simulink model "SEPotencia_ControlTiempoReal_PBL"  (R2021a)
settings: Solver=ode3  StartTime=0.0  StopTime=SimulationTime  FixedStep=StepTime  RelTol=1e-4
PreLoadFcn:
  | clear all;
  | clc;
  | mex Moduladora.c;
  | 
  | %% Parametros Simulacion
  | StepTime = 1.6e-6;
  | SimulationTime = 2;
  | ConstanteTiempo = 159e-6;
  | 
  | %% Motor
  | P = 186.5;
  | Vff = 220;
  | FrecFundamental =  60;
  | VelocidadMotor = 1800;
  | ParPolos = 2;
  | Rs = 11.05;
  | Ls = 3.164e-3;
  | Rr = 6.11;
  | Lr = Ls;
  | Lm = 293.94e-3;
  | Inercia = 0.0005;
  | Tm = 0.05;
  | 
  | %% Consigna Velocidad
  | velocidadInicial=1725/VelocidadMotor;
  | velocidadStepTime = 1;
  | velocidadFinal = 1725/VelocidadMotor;
  | 
  | %% Inversor
  | Vdc = 311;
  | Tconmut = 200e-6;
  | FrecConmut=1/Tconmut;
  | RampaAceleracion = 500/0.2/VelocidadMotor;
  | TiempoMuerto = 4e-6;
  | Kc=1/6;
  | 
  | %% DSP
  | NBits = 12;
  | OffSet = 0.1;
  | PWMSelect = 1; % Pot <= 0, DSP > 0
  | 
  | %Control
  | Kp = 200;
  | Ki = 0;
  | Kd = 0;
  | Control = 1; % Control PI <= 0, Control Step > 0
  | Activar3Armonico = 1; % 3Armonico Activo > 0, 3Armonico Desativado <= 0
  | OverCurrentLimit = 10;
  | VffPU = Vff/Vdc/0.6124;
  | if (Activar3Armonico > 0)
  |     limiteSuperior = 1.154;
  |     if (VffPU > limiteSuperior)
  |         VffPU = limiteSuperior;
  |     end
  | else
  |     limiteSuperior = 1;
  |     if (VffPU > limiteSuperior)
  |         VffPU = limiteSuperior;
  |     end
  | end
  | RelacionVF = (VffPU-0)/(1-0);
  | PI_Num = 3.14159265359;
InitFcn:
  | clear all;
  | clc;
  | mex Moduladora.c;
  | 
  | %% Parametros Simulacion
  | StepTime = 1.6e-6;
  | SimulationTime = 2;
  | ConstanteTiempo = 159e-6;
  | 
  | %% Motor
  | P = 186.5;
  | Vff = 220;
  | FrecFundamental =  60;
  | VelocidadMotor = 1800;
  | ParPolos = 2;
  | Rs = 11.05;
  | Ls = 3.164e-3;
  | Rr = 6.11;
  | Lr = Ls;
  | Lm = 293.94e-3;
  | Inercia = 0.0005;
  | Tm = 0.05;
  | 
  | %% Consigna Velocidad
  | velocidadInicial=600/VelocidadMotor;
  | velocidadStepTime = 1;
  | velocidadFinal = 850/VelocidadMotor;
  | 
  | %% Inversor
  | Vdc = 311;
  | Tconmut = 200e-6;
  | FrecConmut=1/Tconmut;
  | RampaAceleracion = 500/0.2/VelocidadMotor;
  | TiempoMuerto = 4e-6;
  | Kc=1/6;
  | 
  | %% DSP
  | NBits = 12;
  | OffSet = 0.1;
  | PWMSelect = 1; % Pot <= 0, DSP > 0
  | 
  | %Control
  | Kp = 5;
  | Ki = 150;
  | Kd = 0;
  | Control = 1; % Control PI <= 0, Control Step > 0
  | Activar3Armonico = 1; % 3Armonico Activo > 0, 3Armonico Desativado <= 0
  | OverCurrentLimit = 10;
  | VffPU = Vff/Vdc/0.6124;
  | if (Activar3Armonico > 0)
  |     limiteSuperior = 1.154;
  |     if (VffPU > limiteSuperior)
  |         VffPU = limiteSuperior;
  |     end
  | else
  |     limiteSuperior = 1;
  |     if (VffPU > limiteSuperior)
  |         VffPU = limiteSuperior;
  |     end
  | end
  | RelacionVF = (VffPU-0)/(1-0);
  | PI_Num = 3.14159265359;
undefined symbols (not defined in the file or in its folder): DiscIntNeverNeededParam
libraries: spsDCVoltageSourceLib x2, spsFirstOrderFilterLib x2, spsRMSLib x2, spsAsynchronousMachineSIUnitsLib x1, pid_lib x1, spsOnDelayLib x1, spsTriangleGeneratorLib x1, spsGroundLib x1, eeGeneralControl x1, spsTwoLevelConverterLib x1, spsThreePhaseVIMeasurementLib x1, spspowerguiLib x1
settings Model: Creator=The MathWorks, Inc.  LastModifiedBy=Yago
settings SolverCC: AlgebraicLoopSolver=TrustRegion  SolverResetMethod=Robust
settings DataIOCC: ReturnWorkspaceOutputs=off
settings OptimizationCC: LifeSpan=inf
settings DebuggingCC: ReadBeforeWriteMsg=DisableAll  WriteAfterWriteMsg=DisableAll  WriteAfterReadMsg=DisableAll  MultiTaskDSMMsg=none  UnconnectedInputMsg=none  UnconnectedOutputMsg=none  UnconnectedLineMsg=none  SFUnexpectedBacktrackingDiag=warning  SFNoUnconditionalDefaultTransitionDiag=warning  SFExecutionAtInitializationDiag=none  SFMachineParentedDataDiag=warning  ArithmeticOperatorsInVariantConditions=warning
settings ModelReferenceCC: UpdateModelReferenceTargets=IfOutOfDate
settings SFSimCC: SFSimEcho=off  SimUseLocalCustomCode=off  CustomCodeUndefinedFunction=UseInterfaceOnly
settings RTWCC: RTWUseLocalCustomCode=off
settings CodeAppCC: StateflowObjectComments=on
settings GRTTargetCC: TargetLangStandard=C89/C90 (ANSI)
settings ConfigComp: CovMetricSettings=dw  CovSaveCumulativeToWorkspaceVar=on  CovSaveSingleToWorkspaceVar=on  CovExternalEMLEnable=off
settings SimscapeCC: SimscapeNormalizeSystem=off  SimscapeNominalValues={1, 'bar'; 1, 'cm^3/s'; 1, 'bar*kg/s'; 1, 'kJ/kg'; 1, 'kW'; }

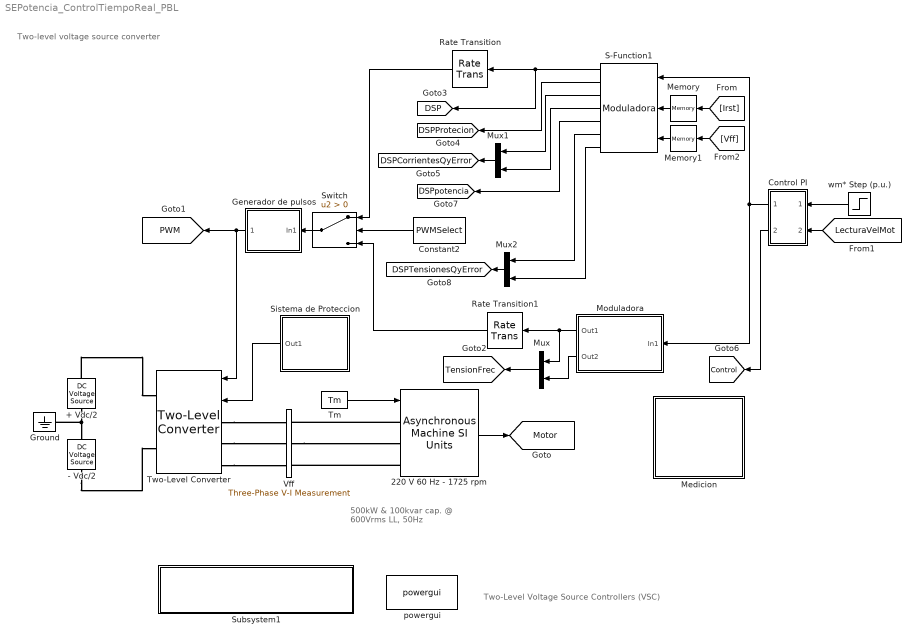
== system SEPotencia_ControlTiempoReal_PBL ==
  note: Two-level voltage source converter
  note: 500kW & 100kvar cap.
      | @ 600Vrms LL, 50Hz
  note: Two-Level Voltage Source Controllers (VSC)
  + Vdc/2 : spsDCVoltageSourceLib/DC Voltage Source  Amplitude=Vdc/2  Measurements=None
  - Vdc/2 : spsDCVoltageSourceLib/DC Voltage Source  Amplitude=Vdc/2  Measurements=None
  220 V 60 Hz - 1725 rpm : spsAsynchronousMachineSIUnitsLib/Asynchronous Machine SI Units  RotorType=Squirrel-cage  PresetModel=No  MechanicalLoad=Torque Tm  ShowDetailedParameters=on  ReferenceFrame=Stationary  Units=SI  MeasurementBus=on  NominalParameters=[ P, Vff, FrecFundamental ]  VoltageRatio=1  Stator="[ Rs  Ls ]"  Rotor="[ Rr  Lr ]"  Cage1=[ 0.022 0.226/377]  Cage2=[ 0.022 0.226/377]  Lm=Lm  Mechanical="[ Inercia  0 ParPolos]"  PolePairs=2  InitialConditions="[ 1,0   0,0,0   0,0,0 ]"  SimulateSaturation=off  Saturation=[14.03593122, 27.81365428, 53.79336849, 72.68890987, 97.98006896, 148.6815601, 215.7428561, 302.9841135, 428.7778367 ; 230, 322, 414, 460, 506, 552, 598, 644, 690]  LoadFlowParameters=0  TsPowergui=0  TsBlock=-1  IterativeModel=Trapezoidal non iterative  IterativeDiscreteModel=Trapezoidal non iterative  Pmec=0
      settings: AttributesFormatString=\n
  Constant2 : Constant  Value=PWMSelect
  Control PI : Subsystem  TreatAsAtomicUnit=on  SystemSampleTime=Tconmut
  Generador de pulsos : Subsystem  SystemSampleTime=Tconmut
  Ground : spsGroundLib/Ground  LConnTagsString=a
  Medicion : Subsystem
  Memory : Memory  LinearizeAsDelay=on
  Memory1 : Memory  LinearizeAsDelay=on
  Moduladora : Subsystem  TreatAsAtomicUnit=on  SystemSampleTime=Tconmut
  Mux : Mux  Inputs=2
  Mux1 : Mux  Inputs=2
  Mux2 : Mux  Inputs=2
  Rate Transition : RateTransition
  Rate Transition1 : RateTransition
  S-Function1 : S-Function  FunctionName=Moduladora  Parameters=Tconmut NBits OffSet RampaAceleracion FrecFundamental FrecConmut Kc limiteSuperior Activar3Armonico OverCurrentLimit Vdc Vff  SFunctionDeploymentMode=off  EnableBusSupport=off
  Sistema de Proteccion : Subsystem
  Subsystem1 : Subsystem  ClipboardFcn=""
      settings: OpenFcn=|
      | t=ScopeData1.time;
      | FundFreq=50;
      | MaxFreq=5000;
      | FFTDATA = power_fftscope(ScopeData1);
      | FFTDATA.input=1;
      | FFTDATA.signal=1;
      | FFTDATA.startTime='last';
      | FFTDATA.cycles=1;
      | FFTDATA.fundamental=FundFreq;
      | FFTDATA.maxFrequency=MaxFreq;
      | FFTDATA.THDmaxFrequency=MaxFreq;
      | FFTDATA.THDbase='fund';
      | power_fftscope(FFTDATA);
      | xlabel('Ia prim 6-pulse');
      | ScreenS=get(0,'Screensize');
      | x0=ScreenS(3); y0=ScreenS(4);
      | PositionParam=[x0/26 y0/3.1 x0/3.8 y0/2.5];
      | set(gcf,'Position',PositionParam);
      | axis([0 5000 0 35])
      | grid
      | FFTDATA = power_fftscope(ScopeData1);
      | FFTDATA.input=3;
      | FFTDATA.signal=1;
      | FFTDATA.startTime='last';
      | FFTDATA.cycles=1;
      | FFTDATA.fundamental=FundFreq;
      | FFTDATA.maxFrequency=MaxFreq;
      | FFTDATA.THDmaxFrequency=MaxFreq;
      | FFTDATA.THDbase='fund';
      | power_fftscope(FFTDATA);
      | xlabel('Ia prim 12-pulse');
      | ScreenS=get(0,'Screensize');
      | x0=ScreenS(3); y0=ScreenS(4);
      | PositionParam=[x0/3.2 y0/3.1 x0/3.8 y0/2.5];
      | set(gcf,'Position',PositionParam);
      | axis([0 5000 0 35])
      | grid
      mask Display: disp('Compare VSC''s\nLine-Line Voltage')
  Switch : Switch  Criteria=u2 > Threshold
  Tm : Constant  Value=Tm
  Two-Level Converter : spsTwoLevelConverterLib/Two-Level Converter  ModelType=Switching devices  Ron=1e-3  Rs=1e6  Cs=inf  Vforward=[0,0]  Ron_Diode=1e-3  Rs_Diode=1e6  Cs_Diode=inf  Vf_Diode=1e-3  Rs_CurrentSource=inf
      settings: SourceProductBaseCode=PS
  Vff : spsThreePhaseVIMeasurementLib/Three-Phase V-I Measurement  VoltageMeasurement=phase-to-phase  SetLabelV=on  LabelV=Vff  Vpu=off  VpuLL=off  CurrentMeasurement=yes  SetLabelI=on  LabelI=Irst  Ipu=off  Pbase=1e3  Vbase=380  OutputType=Magnitude  PhasorSimulation=off  PSBequivalent=0
  powergui : spspowerguiLib/powergui  Priority=1  SimulationMode=Discrete  SampleTime=StepTime  frequency=60  Iterations=50  frequencyindice=0  Pbase=100e6  ErrMax=1e-4  UnitsV=kV  UnitsW=MW  buscounter=0  FunctionMessages=off  echomessages=off  EnableUseOfTLC=off  CurrentSourceSwitches=off  DisableSnubberDevices=off  DisableRonSwitches=off  DisableVfSwitches=off  DisplayEquations=off  AutomaticDiscreteSolvers=off  SolverType=Tustin/Backward Euler (TBE)  Interpol=off  ExternalGateDelay=off  methode=off  Ts=100  x0status=blocks  SPID=off  SwTol=0  HookPort=off  NonlinearTolerance=1e-4  nMaxIteration=100  ContinueOnMaxIteration=off  RestoreLinks=warning  ResistiveCurrentMeasurement=off  Frange=[0:2:500]  Ylog=off  Xlog=on  ShowGrid=off  save=off  variable=ZData  structure=0  ZoomFFT=off  StartTime=0.0  cycles=1  DisplayStyle=1  fundamental=60  FreqAxis=off  MaxFrequency=1000  frequencyindicesteady=1  RmsSteady=1  display=off
  wm* Step (p.u.) : Step  Time=velocidadStepTime  Before=velocidadInicial  After=velocidadFinal  SampleTime=StepTime
  tag scope: Control=global, DSP=global, DSPCorrientesQyError=global, DSPProtecion=global, DSPTensionesQyError=global, DSPpotencia=global, Motor=global, PWM=global, TensionFrec=global
  wires:
  S-Function1/1 -> [DSP], Rate Transition/1
  Constant2/1 -> Switch/2
  Memory/1 -> S-Function1/2
  Tm/1 -> 220 V 60 Hz - 1725 rpm/1
  220 V 60 Hz - 1725 rpm/1 -> [Motor]
  Rate Transition/1 -> Switch/1
  Switch/1 -> Generador de pulsos/1(In1)
  Moduladora/1(Out1) -> Rate Transition1/1, Mux/1
  Generador de pulsos/1("  ") -> [PWM], Two-Level Converter/1
  Mux/1 -> [TensionFrec]
  Moduladora/2(Out2) -> Mux/2
  Rate Transition1/1 -> Switch/3
  S-Function1/2 -> [DSPProtecion]
  Control PI/1(Out1) -> S-Function1/1, Moduladora/1(In1)
  wm* Step (p.u.)/1 -> Control PI/1(In1)
  Sistema de Proteccion/1(Out1) -> Two-Level Converter/2
  Mux1/1 -> [DSPCorrientesQyError]
  S-Function1/3 -> Mux1/1
  S-Function1/4 -> Mux1/2
  [Irst] -> Memory/1
  [LecturaVelMot] -> Control PI/2(In2)
  Control PI/2(Out2) -> [Control]
  [Vff] -> Memory1/1
  Memory1/1 -> S-Function1/3
  S-Function1/5 -> [DSPpotencia]
  S-Function1/6 -> Mux2/1
  S-Function1/7 -> Mux2/2
  Mux2/1 -> [DSPTensionesQyError]
  connections:
  Two-Level Converter/LConn2 -- Vff/LConn2
  220 V 60 Hz - 1725 rpm/LConn3 -- Vff/RConn3
  Two-Level Converter/LConn3 -- Vff/LConn3
  Two-Level Converter/LConn1 -- Vff/LConn1
  220 V 60 Hz - 1725 rpm/LConn1 -- Vff/RConn1
  + Vdc/2/RConn1 -- Two-Level Converter/RConn1
  - Vdc/2/LConn1 -- Two-Level Converter/RConn2
  + Vdc/2/LConn1 -- - Vdc/2/RConn1 -- Ground/LConn1
  Vff/RConn2 -- 220 V 60 Hz - 1725 rpm/LConn2

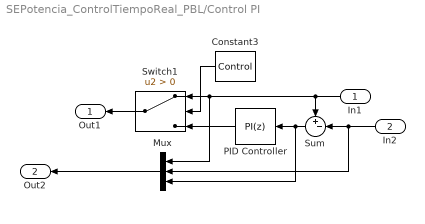
== system SEPotencia_ControlTiempoReal_PBL/Control PI ==
  In1 : Inport
  In2 : Inport  Port=2
  Constant3 : Constant  Value=Control
  Mux : Mux  Inputs=3
  PID Controller : pid_lib/PID Controller  Controller=PI  Form=Parallel  TimeDomain=Discrete-time  UseExternalTs=off  SampleTime=-1  IntegratorMethod=Trapezoidal  FilterMethod=Forward Euler  ControllerParametersSource=internal  P=Kp  I=1/Ki  D=Kd  UseFilter=on  N=100  TunerSelectOption=Transfer Function Based (PID Tuner App)  InitialConditionSource=internal  InitialConditionForIntegrator=0  InitialConditionForFilter=0  DifferentiatorICPrevScaledInput=0  ExternalReset=none  TrackingMode=off  Kt=1  LimitOutput=on  SatLimitsSource=internal  UpperSaturationLimit=1.5  LowerSaturationLimit=-1.5  LinearizeAsGain=on  AntiWindupMode=none  Kb=1  POutMin=[]  POutMax=[]  IOutMin=[]  IOutMax=[]  DOutMin=[]  DOutMax=[]  NOutMin=[]  NOutMax=[]  SumOutMin=[]  SumOutMax=[]  SaturationOutMin=[]  SaturationOutMax=[]  PParamMin=[]  PParamMax=[]  IParamMin=[]  IParamMax=[]  DParamMin=[]  DParamMax=[]  NParamMin=[]  NParamMax=[]  KbParamMin=[]  KbParamMax=[]  KtParamMin=[]  KtParamMax=[]  KbOutMin=[]  KbOutMax=[]  KtOutMin=[]  KtOutMax=[]  IntegratorOutMin=[]  IntegratorOutMax=[]  FilterOutMin=[]  FilterOutMax=[]  SumI1OutMin=[]  SumI1OutMax=[]  SumI2OutMin=[]  SumI2OutMax=[]  SumI3OutMin=[]  SumI3OutMax=[]  SumI4OutMin=[]  SumI4OutMax=[]  SumDOutMin=[]  SumDOutMax=[]  DifferentiatorOutMin=[]  DifferentiatorOutMax=[]  FilterDiffOutCoefMin=[]  FilterDiffOutCoefMax=[]  ReciprocalOutMin=[]  ReciprocalOutMax=[]  SumDenOutMin=[]  SumDenOutMax=[]  SumNumOutMin=[]  SumNumOutMax=[]  DivideOutMin=[]  DivideOutMax=[]  UdiffTsProdOutMin=[]  UdiffTsProdOutMax=[]  NTsProdOutMin=[]  NTsProdOutMax=[]  UintegralTsProdOutMin=[]  UintegralTsProdOutMax=[]  UngainTsProdOutMin=[]  UngainTsProdOutMax=[]  IntegratorContinuousStateAttributes=''  IntegratorStateMustResolveToSignalObject=off  IntegratorRTWStateStorageClass=Auto  FilterContinuousStateAttributes=''  FilterStateMustResolveToSignalObject=off  FilterRTWStateStorageClass=Auto  ParallelPVariant=InternalParameters  IdealPVariant=Disabled  IVariant=InternalParameters  DVariant=Disabled  IntegratorVariant=Discrete  SatVariant=Enabled  AWVariant=Passthrough  PCopyVariant=Disabled  TRVariant=Disabled  FdbkBlocksVariant=Forward  IdealPFdbkVariant=Disabled  SatFdbkVariant=Disabled  DerivativeFilterVariant=Disabled  NVariant=Disabled  NCopyVariant=Disabled_SignalSpec  FilterICVariant=Disabled  IntegratorICVariant=InternalICs  ExternalResetVariant=Disabled  TRSumVariant=Passthrough  SumFdbkVariant=Disabled  SumVariant=Sum_PI  TsampFilterVariant=InternalTs  TsampNgainVariant=Passthrough  TsampIntegralVariant=Passthrough  ExternalSaturationOutDataTypeStr=Inherit: Same as second input
  Sum : Sum  Inputs=+-|
  Switch1 : Switch  Criteria=u2 > Threshold
  Out1 : Outport
  Out2 : Outport  Port=2
  wires:
  In1/1 -> Mux/1, Switch1/1, Sum/1
  PID Controller/1 -> Switch1/3
  Sum/1 -> Mux/3, PID Controller/1
  Constant3/1 -> Switch1/2
  Switch1/1 -> Out1/1
  In2/1 -> Mux/2, Sum/2
  Mux/1 -> Out2/1

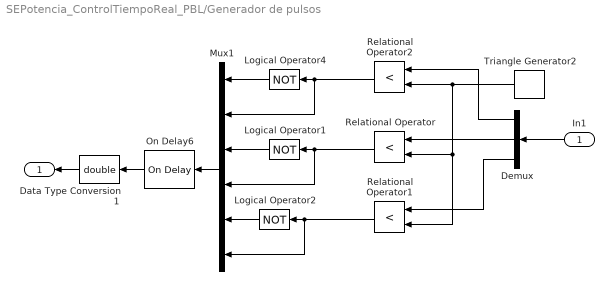
== system SEPotencia_ControlTiempoReal_PBL/Generador de pulsos ==
  In1 : Inport
  Data Type Conversion1 : DataTypeConversion  OutDataTypeStr=double
  Demux : Demux  Outputs=3
  Logical Operator1 : Logic  Operator=NOT
  Logical Operator2 : Logic  Operator=NOT
  Logical Operator4 : Logic  Operator=NOT
  Mux1 : Mux  Inputs=6
  On Delay6 : spsOnDelayLib/On Delay  DelayType=On delay  delay=TiempoMuerto  ic=0  Ts=0
      settings: SourceProductBaseCode=PS
  Relational Operator : RelationalOperator  Operator=<  OutDataTypeStr=boolean  RndMeth=Simplest
  Relational Operator1 : RelationalOperator  Operator=<  OutDataTypeStr=boolean  RndMeth=Simplest
  Relational Operator2 : RelationalOperator  Operator=<  OutDataTypeStr=boolean  RndMeth=Simplest
  Triangle Generator2 : spsTriangleGeneratorLib/Triangle Generator  Freq=FrecConmut  Phase=90  Ts=StepTime
  "  " : Outport
  wires:
  Logical Operator2/1 -> Mux1/5
  Data Type Conversion1/1 -> "  "/1
  Logical Operator1/1 -> Mux1/3
  Mux1/1 -> On Delay6/1
  Relational Operator1/1 -> Mux1/6, Logical Operator2/1
  Relational Operator/1 -> Mux1/4, Logical Operator1/1
  Logical Operator4/1 -> Mux1/1
  Relational Operator2/1 -> Mux1/2, Logical Operator4/1
  Demux/1 -> Relational Operator2/1
  Demux/2 -> Relational Operator/1
  Triangle Generator2/1 -> Relational Operator1/2, Relational Operator/2, Relational Operator2/2
  Demux/3 -> Relational Operator1/1
  In1/1 -> Demux/1
  On Delay6/1 -> Data Type Conversion1/1

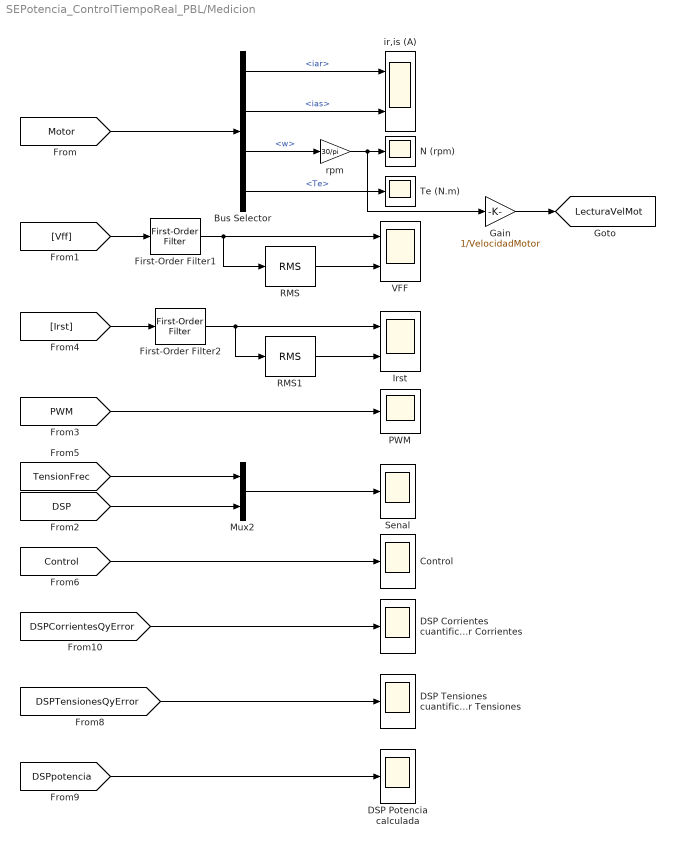
== system SEPotencia_ControlTiempoReal_PBL/Medicion ==
  Bus Selector : BusSelector  OutputSignals=iar,ias,w,Te
  Control : Scope
  DSP Corrientes cuantificadas y Error Corrientes : Scope
  DSP Potencia calculada : Scope
  DSP Tensiones cuantificadas y Error Tensiones : Scope
  First-Order Filter1 : spsFirstOrderFilterLib/First-Order Filter  FilterType=Lowpass  Tc=ConstanteTiempo  Ts=StepTime  Initialize=on  Vac_Init=[0, 0, 60]  Vdc_Init=0  PlotResponse=off  FreqRange="[0,  200,  1]"
  First-Order Filter2 : spsFirstOrderFilterLib/First-Order Filter  FilterType=Lowpass  Tc=ConstanteTiempo  Ts=StepTime  Initialize=on  Vac_Init=[0, 0, 60]  Vdc_Init=0  PlotResponse=off  FreqRange="[0,  200,  1]"
  Gain : Gain  Gain=1/VelocidadMotor
  Irst : Scope  NumInputPorts=2
  Mux2 : Mux  Inputs=2
  N (rpm) : Scope
  PWM : Scope
  RMS : spsRMSLib/RMS  TrueRMS=on  Freq=FrecFundamental*velocidadFinal  RMSInit=0  Ts=StepTime
  RMS1 : spsRMSLib/RMS  TrueRMS=on  Freq=FrecFundamental*velocidadFinal  RMSInit=0  Ts=StepTime
  Senal : Scope
  Te (N.m) : Scope
  VFF : Scope  NumInputPorts=2
  ir,is (A) : Scope  NumInputPorts=2
  rpm : Gain  Gain=30/pi  SaturateOnIntegerOverflow=on  OutDataTypeStr=Inherit: Same as input  ParamDataTypeStr=Inherit: Same as input
  tag scope: LecturaVelMot=global
  wires:
  Mux2/1 -> Senal/1
  [Vff] -> First-Order Filter1/1
  [DSP] -> Mux2/2
  First-Order Filter1/1 -> RMS/1, VFF/1
  RMS1/1 -> Irst/2
  [Motor] -> Bus Selector/1
  [Irst] -> First-Order Filter2/1
  [TensionFrec] -> Mux2/1
  Bus Selector/3 -> rpm/1  "<w>"
  First-Order Filter2/1 -> RMS1/1, Irst/1
  RMS/1 -> VFF/2
  Bus Selector/1 -> ir,is (A)/1  "<iar>"
  [PWM] -> PWM/1
  Bus Selector/4 -> Te (N.m)/1  "<Te>"
  rpm/1 -> Gain/1, N (rpm)/1
  Bus Selector/2 -> ir,is (A)/2  "<ias>"
  Gain/1 -> [LecturaVelMot]
  [Control] -> Control/1
  [DSPTensionesQyError] -> DSP Tensiones cuantificadas y Error Tensiones/1
  [DSPpotencia] -> DSP Potencia calculada/1
  [DSPCorrientesQyError] -> DSP Corrientes cuantificadas y Error Corrientes/1

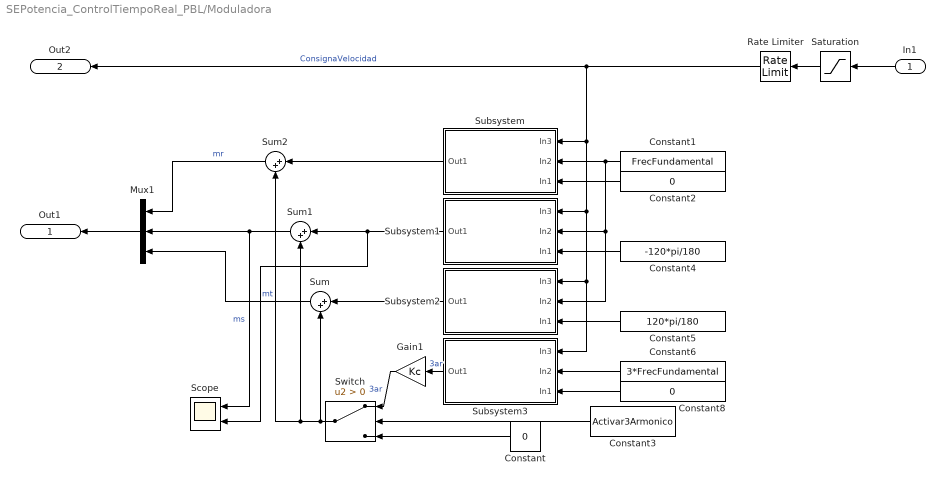
== system SEPotencia_ControlTiempoReal_PBL/Moduladora ==
  In1 : Inport
  Constant : Constant  Value=0
  Constant1 : Constant  Value=FrecFundamental
  Constant2 : Constant  Value=0
  Constant3 : Constant  Value=Activar3Armonico
  Constant4 : Constant  Value=-120*pi/180
  Constant5 : Constant  Value=120*pi/180
  Constant6 : Constant  Value=3*FrecFundamental
  Constant8 : Constant  Value=0
  Gain1 : Gain  Gain=Kc
  Mux1 : Mux  Inputs=3
  Rate Limiter : RateLimiter  RisingSlewLimit=RampaAceleracion  FallingSlewLimit=-RampaAceleracion  SampleTimeMode=inherited
  Saturation : Saturate  UpperLimit=1  LowerLimit=OffSet
  Scope : Scope  NumInputPorts=2
  Subsystem : Subsystem
  Subsystem1 : Subsystem
  Subsystem2 : Subsystem
  Subsystem3 : Subsystem
  Sum : Sum  Inputs=|++
  Sum1 : Sum  Inputs=|++
  Sum2 : Sum  Inputs=|++
  Switch : Switch  Criteria=u2 > Threshold
  Out1 : Outport
  Out2 : Outport  Port=2
  wires:
  Constant1/1 -> Subsystem/2(In2), Subsystem2/2(In2), Subsystem1/2(In2)
  Constant6/1 -> Subsystem3/2(In2)
  In1/1 -> Saturation/1
  Subsystem/1(Out1) -> Sum2/1
  Constant4/1 -> Subsystem1/3(In1)
  Subsystem2/1(Out1) -> Sum/1
  Constant2/1 -> Subsystem/3(In1)
  Constant5/1 -> Subsystem2/3(In1)
  Constant8/1 -> Subsystem3/3(In1)
  Subsystem1/1(Out1) -> Scope/2, Sum1/1
  Rate Limiter/1 -> Subsystem1/1(In3), Subsystem3/1(In3), Subsystem2/1(In3), Subsystem/1(In3), Out2/1  "ConsignaVelocidad"
  Saturation/1 -> Rate Limiter/1
  Gain1/1 -> Switch/1  "3ar"
  Constant/1 -> Switch/3
  Switch/1 -> Sum2/2, Sum1/2, Sum/2
  Sum/1 -> Mux1/3  "mt"
  Sum1/1 -> Scope/1, Mux1/2  "ms"
  Sum2/1 -> Mux1/1  "mr"
  Mux1/1 -> Out1/1
  Constant3/1 -> Switch/2
  Subsystem3/1(Out1) -> Gain1/1  "3ar"

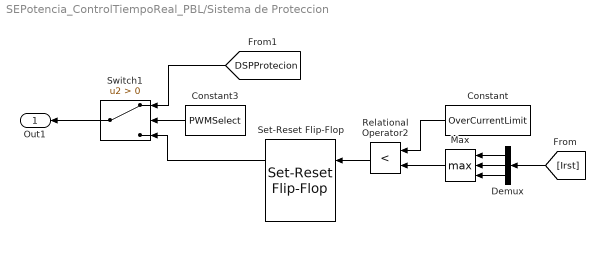
== system SEPotencia_ControlTiempoReal_PBL/Sistema de Proteccion ==
  Constant : Constant  Value=OverCurrentLimit
  Constant3 : Constant  Value=PWMSelect
  Demux : Demux  Outputs=3
  Max : MinMax  Function=max  Inputs=3
  Relational Operator2 : RelationalOperator  Operator=<  OutDataTypeStr=boolean  RndMeth=Simplest
  Set-Reset Flip-Flop : eeGeneralControl/Set-Reset Flip-Flop  LabelModeActiveChoice=Discrete  UndefState=Set  Q0=0  Ts=-1
      settings: SourceProductBaseCode=PS
  Switch1 : Switch  Criteria=u2 > Threshold
  Out1 : Outport
  wires:
  Constant3/1 -> Switch1/2
  Constant/1 -> Relational Operator2/1
  Set-Reset Flip-Flop/1 -> Switch1/3
  Relational Operator2/1 -> Set-Reset Flip-Flop/1
  [DSPProtecion] -> Switch1/1
  [Irst] -> Demux/1
  Switch1/1 -> Out1/1
  Demux/1 -> Max/1
  Demux/2 -> Max/2
  Demux/3 -> Max/3
  Max/1 -> Relational Operator2/2

== system SEPotencia_ControlTiempoReal_PBL/Subsystem1 ==

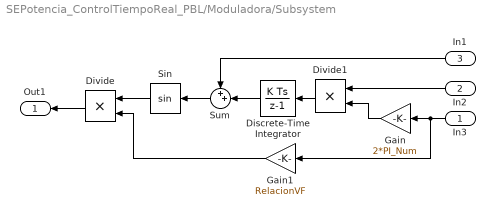
== system SEPotencia_ControlTiempoReal_PBL/Moduladora/Subsystem ==
  In3 : Inport
  In2 : Inport  Port=2
  In1 : Inport  Port=3
  Discrete-Time Integrator : DiscreteIntegrator  SampleTime=Tconmut  ICPrevOutput=DiscIntNeverNeededParam  ICPrevScaledInput=DiscIntNeverNeededParam
  Divide : Product  Inputs=**
  Divide1 : Product  Inputs=**
  Gain : Gain  Gain=2*PI_Num
  Gain1 : Gain  Gain=RelacionVF
  Sin : Trigonometry
  Sum : Sum  Inputs=++|
  Out1 : Outport
  wires:
  In3/1 -> Gain/1, Gain1/1
  Sin/1 -> Divide/1
  Gain/1 -> Divide1/2
  In2/1 -> Divide1/1
  Divide/1 -> Out1/1
  Divide1/1 -> Discrete-Time Integrator/1
  Sum/1 -> Sin/1
  In1/1 -> Sum/1
  Discrete-Time Integrator/1 -> Sum/2
  Gain1/1 -> Divide/2

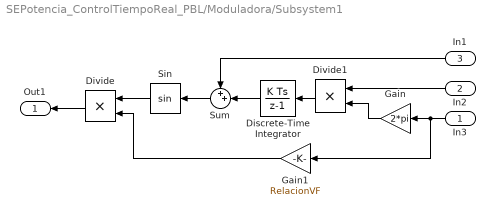
== system SEPotencia_ControlTiempoReal_PBL/Moduladora/Subsystem1 ==
  In3 : Inport
  In2 : Inport  Port=2
  In1 : Inport  Port=3
  Discrete-Time Integrator : DiscreteIntegrator  SampleTime=Tconmut  ICPrevOutput=DiscIntNeverNeededParam  ICPrevScaledInput=DiscIntNeverNeededParam
  Divide : Product  Inputs=**
  Divide1 : Product  Inputs=**
  Gain : Gain  Gain=2*pi
  Gain1 : Gain  Gain=RelacionVF
  Sin : Trigonometry
  Sum : Sum  Inputs=++|
  Out1 : Outport
  wires:
  Discrete-Time Integrator/1 -> Sum/2
  In1/1 -> Sum/1
  Sum/1 -> Sin/1
  Divide1/1 -> Discrete-Time Integrator/1
  Divide/1 -> Out1/1
  In2/1 -> Divide1/1
  Gain/1 -> Divide1/2
  Sin/1 -> Divide/1
  In3/1 -> Gain1/1, Gain/1
  Gain1/1 -> Divide/2

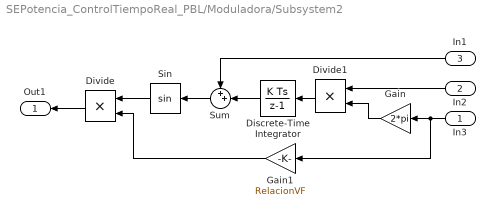
== system SEPotencia_ControlTiempoReal_PBL/Moduladora/Subsystem2 ==
  In3 : Inport
  In2 : Inport  Port=2
  In1 : Inport  Port=3
  Discrete-Time Integrator : DiscreteIntegrator  SampleTime=Tconmut  ICPrevOutput=DiscIntNeverNeededParam  ICPrevScaledInput=DiscIntNeverNeededParam
  Divide : Product  Inputs=**
  Divide1 : Product  Inputs=**
  Gain : Gain  Gain=2*pi
  Gain1 : Gain  Gain=RelacionVF
  Sin : Trigonometry
  Sum : Sum  Inputs=++|
  Out1 : Outport
  wires:
  In3/1 -> Gain/1, Gain1/1
  Sin/1 -> Divide/1
  Gain/1 -> Divide1/2
  In2/1 -> Divide1/1
  Divide/1 -> Out1/1
  Divide1/1 -> Discrete-Time Integrator/1
  Sum/1 -> Sin/1
  In1/1 -> Sum/1
  Discrete-Time Integrator/1 -> Sum/2
  Gain1/1 -> Divide/2

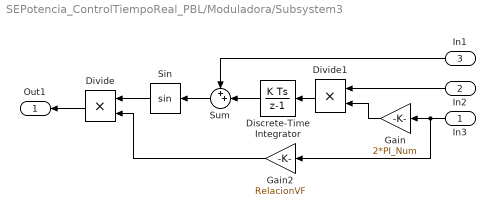
== system SEPotencia_ControlTiempoReal_PBL/Moduladora/Subsystem3 ==
  In3 : Inport
  In2 : Inport  Port=2
  In1 : Inport  Port=3
  Discrete-Time Integrator : DiscreteIntegrator  SampleTime=Tconmut  ICPrevOutput=DiscIntNeverNeededParam  ICPrevScaledInput=DiscIntNeverNeededParam
  Divide : Product  Inputs=**
  Divide1 : Product  Inputs=**
  Gain : Gain  Gain=2*PI_Num
  Gain2 : Gain  Gain=RelacionVF
  Sin : Trigonometry
  Sum : Sum  Inputs=++|
  Out1 : Outport
  wires:
  Discrete-Time Integrator/1 -> Sum/2
  In1/1 -> Sum/1
  Sum/1 -> Sin/1
  Divide1/1 -> Discrete-Time Integrator/1
  Divide/1 -> Out1/1
  In2/1 -> Divide1/1
  Gain/1 -> Divide1/2
  Sin/1 -> Divide/1
  In3/1 -> Gain2/1, Gain/1
  Gain2/1 -> Divide/2
